simulink model "SimulinkTemperatura"  (R2022b)
settings: Solver=FixedStepAuto  StartTime=0.0  StopTime=1200  FixedStep=0.5  RelTol=1e-3
values from neighbouring files (symbols this model uses):
  A = [-1 1; 0 0]    [Tiempos.m]    (also in temperatura.m)
  B = [0 1; 1 0]    [Tiempos.m]    (also in temperatura.m)
  C = [1 0; 0 1]    [Tiempos.m]    (also in temperatura.m)
  CL = 0    [Tiempos.m]    (also in temperatura.m)
  D = [0 0; 0 0]    [Tiempos.m]    (also in temperatura.m)
  T0 = 25    [Tiempos.m]    (also in temperatura.m)
  Ta = 25    [Tiempos.m]    (also in temperatura.m)
  Tobj = Tobjs(i)    [Tiempos.m]    (also in temperatura.m = 20)
libraries: mpclib x1, simulink x1
settings Model: Creator=Usuario  LastModifiedBy=Usuario

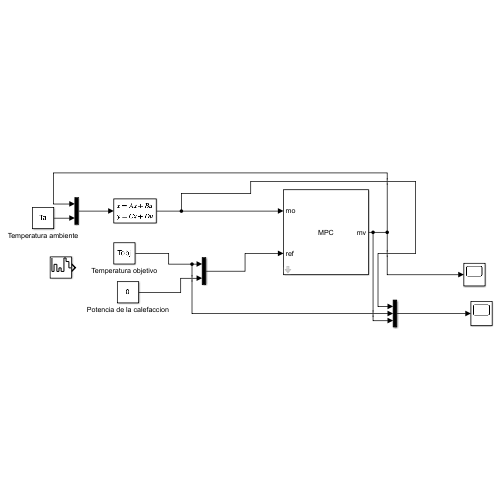
[thumbnail: Simulink's stored preview of the top-level diagram]
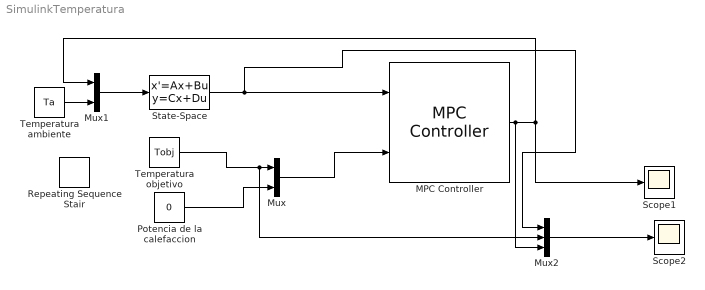
== system SimulinkTemperatura ==
  MPC Controller : mpclib/MPC Controller  SCDEnableBlockLinearizationSpecification=on  mpcobj=mpc_temperatura  is_multiple=0  enable_value=0  return_u0=off  updateMPCinCallerWorkspace=on  md_inport=off  mv_inport=off  uref_inport=off  return_cost=off  return_mvseq=off  return_qpstatus=off  return_xseq=off  return_state=off  return_ovseq=off  state_inport=off  umin_inport=off  umax_inport=off  ymin_inport=off  ymax_inport=off  cc_inport=off  ywt_inport=off  uwt_inport=off  duwt_inport=off  rhoeps_inport=off  pm_inport=off  MaximumP=10  HorizonChoice=FixedHorizon  n_ts=0.5  n_p=120  n_mv=1  n_md=0  n_ud=1  n_mo=2  n_uo=0  BlockDataType=double  SampleTimeInherited=off  switch_inport=off
  Mux : Mux  Inputs=2
  Mux1 : Mux  Inputs=2
  Mux2 : Mux  Inputs=3
  Potencia de la calefaccion : Constant  Value=0
  Repeating Sequence Stair : simulink/Sources/Repeating Sequence Stair  OutValues="[20 22  20 21 20 24 23 21].'"  tsamp=150  OutMin=[]  OutMax=[]  OutDataTypeStr=double  OutputDataTypeScalingMode=double  OutDataType=fixdt(0,8)  ConRadixGroup=Best Precision: Vector-wise  OutScaling=2^-12
  Scope1 : Scope
  Scope2 : Scope
  State-Space : StateSpace  A=A  B=B  C=C  D=D  InitialCondition=[T0;CL]  ParameterTunability=Optimized
  Temperatura ambiente : Constant  Value=Ta
  Temperatura objetivo : Constant  Value=Tobj
  wires:
  MPC Controller/1 -> Mux2/3, Scope1/1, Mux1/1
  Potencia de la calefaccion/1 -> Mux/2
  Mux/1 -> MPC Controller/2
  Mux1/1 -> State-Space/1
  Temperatura ambiente/1 -> Mux1/2
  State-Space/1 -> Mux2/1, MPC Controller/1
  Mux2/1 -> Scope2/1
  Temperatura objetivo/1 -> Mux2/2, Mux/1
